simulink model "hexarotor_dynamic_model"  (Simulink 8.5)
settings: Solver=ode45  StartTime=0.0  StopTime=20  RelTol=1e-3
libraries: aerolib6dof2 x1
settings Model: Creator=flying  LastModifiedBy=flying
settings DataIOCC: ExternalInput=getinputstruct(op_trim1)  InitialState=getstatestruct(op_trim1)  LoadExternalInput=on  LoadInitialState=on  SignalLoggingSaveFormat=Dataset
settings OptimizationCC: ExpressionDepthLimit=128
settings DebuggingCC: UnderspecifiedInitializationDetection=Simplified  MergeDetectMultiDrivingBlocksExec=error  FcnCallInpInsideContextMsg=EnableAllAsError  StateNameClashWarn=none
settings GRTTargetCC: CombineOutputUpdateFcns=on  GRTInterface=off

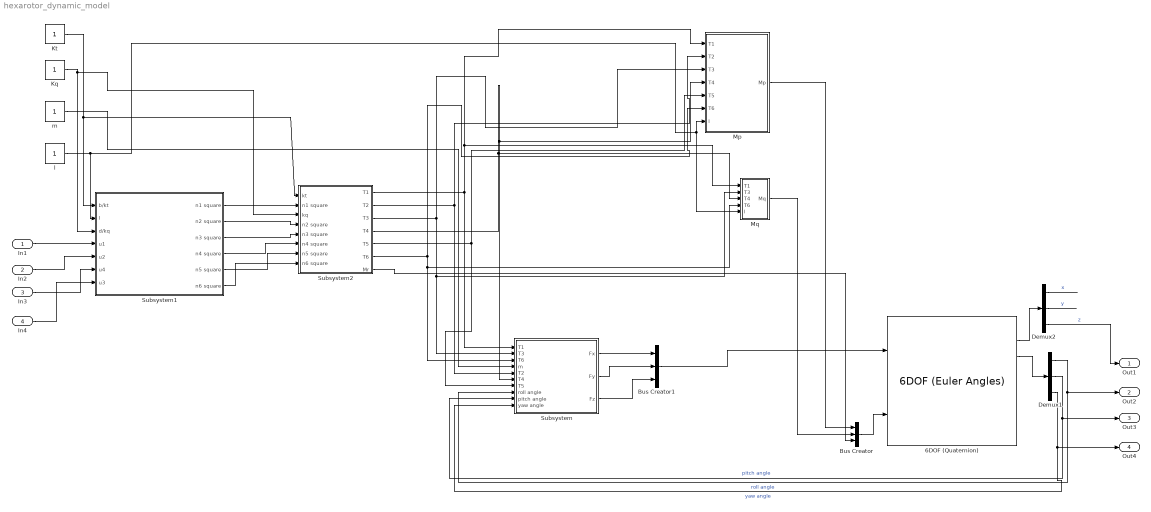
== system hexarotor_dynamic_model ==
  In1 : Inport
  In2 : Inport  Port=2
  In3 : Inport  Port=3
  In4 : Inport  Port=4
  6DOF (Quaternion) : aerolib6dof2/6DOF (Euler Angles)  units=Metric (MKS)  mtype=Fixed  rep=Quaternion  xme_0=[0 0 0]  Vm_0=[0 0 0]  eul_0=[0 0 0]  pm_0=[0 0 0]  mass_0=1.0  mass_e=0.5  mass_f=2.0  inertia=eye(3)  inertia_e=eye(3)  inertia_f=2*eye(3)  k_quat=1.0  vre_flag=on
  Bus Creator : BusCreator  Inputs=3
  Bus Creator1 : BusCreator  Inputs=3
  Demux1 : Demux  Outputs=3
  Demux2 : Demux  Outputs=3
  Kq : Constant
  Kt : Constant
  Mp : Subsystem
  Mq : Subsystem
  Subsystem : Subsystem
  Subsystem1 : Subsystem
  Subsystem2 : Subsystem
  l : Constant
  m : Constant
  Out1 : Outport
  Out2 : Outport  Port=2
  Out3 : Outport  Port=3
  Out4 : Outport  Port=4
  wires:
  6DOF (Quaternion)/3 -> Demux1/1
  l/1 -> Subsystem1/2(l), Mq/5(l), Mp/7(l)
  Mp/1(Mp) -> Bus Creator/1
  Mq/1(Mq) -> Bus Creator/2
  Subsystem2/2(T2) -> Mp/2(T2), Subsystem/5(T2)
  Subsystem2/4(T4) -> Subsystem/6(T4), Mp/4(T4), Mq/3(T4)
  Subsystem2/1(T1) -> Mp/1(T1), Mq/1(T1), Subsystem/1(T1)
  Subsystem2/6(T6) -> Subsystem/3(T6), Mq/4(T6), Mp/6(T6)
  Subsystem2/3(T3) -> Subsystem/2(T3), Mq/2(T3), Mp/3(T3)
  Subsystem2/5(T5) -> Subsystem/7(T5), Mp/5(T5)
  Kt/1 -> Subsystem1/1(b/kt), Subsystem2/1(kt)
  Kq/1 -> Subsystem1/3(d/kq), Subsystem2/3(kq)
  Subsystem2/7(Mr) -> Bus Creator/3
  Bus Creator/1 -> 6DOF (Quaternion)/2
  m/1 -> Subsystem/4(m)
  Demux1/1 -> Out2/1, Subsystem/8(roll angle)  "roll angle"
  Demux1/2 -> Out3/1, Subsystem/9(pitch angle)  "pitch angle"
  Demux1/3 -> Out4/1, Subsystem/10(yaw angle)  "yaw angle"
  Subsystem/1(Fx) -> Bus Creator1/1
  Subsystem/2(Fy) -> Bus Creator1/2
  Subsystem/3(Fz) -> Bus Creator1/3
  Bus Creator1/1 -> 6DOF (Quaternion)/1
  Subsystem1/1(n1 square) -> Subsystem2/2(n1 square)
  Subsystem1/2(n2 square) -> Subsystem2/4(n2 square)
  Subsystem1/3(n3 square) -> Subsystem2/5(n3 square)
  Subsystem1/4(n4 square) -> Subsystem2/6(n4 square)
  Subsystem1/5(n5 square) -> Subsystem2/7(n5 square)
  Subsystem1/6(n6 square) -> Subsystem2/8(n6 square)
  6DOF (Quaternion)/2 -> Demux2/1
  Demux2/1 -> ?  "x"
  Demux2/2 -> ?  "y"
  Demux2/3 -> Out1/1  "z"
  In1/1 -> Subsystem1/4(u1)
  In2/1 -> Subsystem1/5(u2)
  In3/1 -> Subsystem1/6(u4)
  In4/1 -> Subsystem1/7(u3)

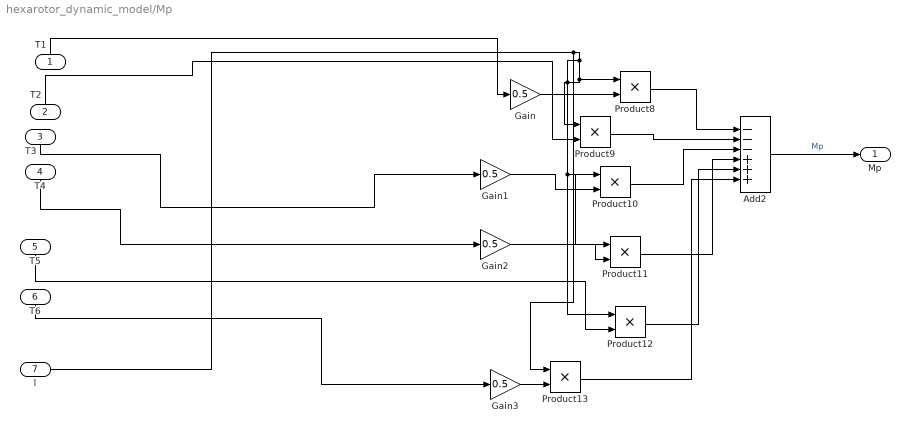
== system hexarotor_dynamic_model/Mp ==
  T1 : Inport
  T2 : Inport  Port=2
  T3 : Inport  Port=3
  T4 : Inport  Port=4
  T5 : Inport  Port=5
  T6 : Inport  Port=6
  l : Inport  Port=7
  Add2 : Sum  Inputs=---+++
  Gain{,1..3} (4 alike) : Gain  Gain=0.5
  Product{8..13} (6 alike) : Product
  Mp : Outport
  wires:
  T5/1 -> Product12/2
  T1/1 -> Gain/1
  T3/1 -> Gain1/1
  T6/1 -> Gain3/1
  T2/1 -> Product9/2
  T4/1 -> Gain2/1
  Add2/1 -> Mp/1  "Mp"
  Product9/1 -> Add2/2
  Product8/1 -> Add2/1
  Product10/1 -> Add2/3
  Gain3/1 -> Product13/2
  Product13/1 -> Add2/6
  Gain1/1 -> Product10/2
  Gain/1 -> Product8/2
  l/1 -> Product13/1, Product12/1, Product11/1, Product10/1, Product9/1, Product8/1
  Product12/1 -> Add2/5
  Gain2/1 -> Product11/2
  Product11/1 -> Add2/4

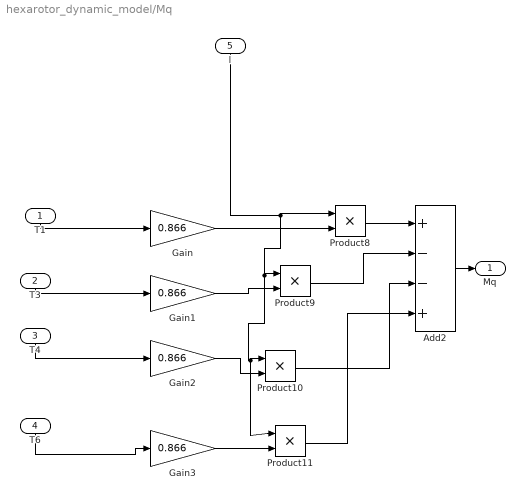
== system hexarotor_dynamic_model/Mq ==
  T1 : Inport
  T3 : Inport  Port=2
  T4 : Inport  Port=3
  T6 : Inport  Port=4
  l : Inport  Port=5
  Add2 : Sum  Inputs=+--+
  Gain{,1..3} (4 alike) : Gain  Gain=0.866
  Product{8..11} (4 alike) : Product
  Mq : Outport
  wires:
  Gain2/1 -> Product10/2
  Gain/1 -> Product8/2
  Gain1/1 -> Product9/2
  Product9/1 -> Add2/2
  Product10/1 -> Add2/3
  Product8/1 -> Add2/1
  Product11/1 -> Add2/4
  Gain3/1 -> Product11/2
  T1/1 -> Gain/1
  l/1 -> Product11/1, Product10/1, Product9/1, Product8/1
  T3/1 -> Gain1/1
  T6/1 -> Gain3/1
  Add2/1 -> Mq/1
  T4/1 -> Gain2/1

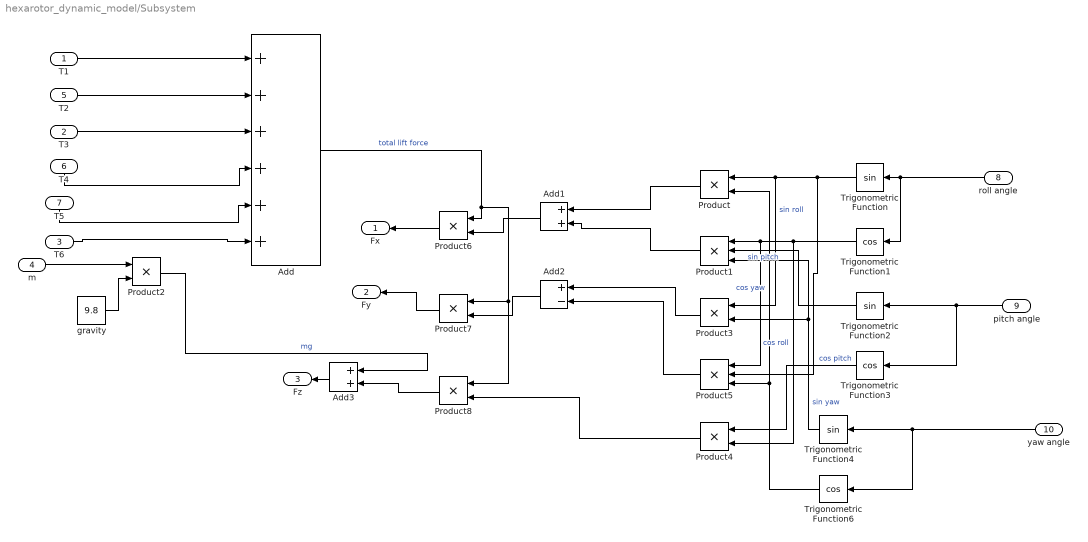
== system hexarotor_dynamic_model/Subsystem ==
  T1 : Inport
  T3 : Inport  Port=2
  T6 : Inport  Port=3
  m : Inport  Port=4
  T2 : Inport  Port=5
  T4 : Inport  Port=6
  T5 : Inport  Port=7
  roll angle : Inport  Port=8
  pitch angle : Inport  Port=9
  yaw angle : Inport  Port=10
  Add : Sum  Inputs=++++++
  Add1 : Sum
  Add2 : Sum  Inputs=+-
  Add3 : Sum
  Product{,2..4,6..8} (7 alike) : Product
  Product1 : Product  Inputs=3
  Product5 : Product  Inputs=3
  Trigonometric Function : Trigonometry
  Trigonometric Function1 : Trigonometry  Operator=cos
  Trigonometric Function2 : Trigonometry
  Trigonometric Function3 : Trigonometry  Operator=cos
  Trigonometric Function4 : Trigonometry
  Trigonometric Function6 : Trigonometry  Operator=cos
  gravity : Constant  Value=9.8
  Fx : Outport
  Fy : Outport  Port=2
  Fz : Outport  Port=3
  wires:
  Product7/1 -> Fy/1
  Product2/1 -> Add3/1  "mg"
  Trigonometric Function6/1 -> Product/2, Product5/3  "cos yaw"
  Product8/1 -> Add3/2
  Trigonometric Function/1 -> Product5/2, Product3/1, Product/1  "sin roll"
  Product1/1 -> Add1/2
  Product/1 -> Add1/1
  Trigonometric Function1/1 -> Product4/2, Product5/1, Product1/1  "cos roll"
  Trigonometric Function4/1 -> Product3/2, Product1/3  "sin yaw"
  Add2/1 -> Product7/2
  Add1/1 -> Product6/2
  Trigonometric Function2/1 -> Product1/2  "sin pitch"
  Product4/1 -> Product8/2
  Product3/1 -> Add2/1
  Product5/1 -> Add2/2
  Add/1 -> Product8/1, Product7/1, Product6/1  "total lift force"
  T1/1 -> Add/1
  T2/1 -> Add/2
  T6/1 -> Add/6
  T5/1 -> Add/5
  Add3/1 -> Fz/1
  T3/1 -> Add/3
  T4/1 -> Add/4
  yaw angle/1 -> Trigonometric Function6/1, Trigonometric Function4/1
  gravity/1 -> Product2/2
  m/1 -> Product2/1
  Product6/1 -> Fx/1
  Trigonometric Function3/1 -> Product4/1  "cos pitch"
  pitch angle/1 -> Trigonometric Function3/1, Trigonometric Function2/1
  roll angle/1 -> Trigonometric Function1/1, Trigonometric Function/1

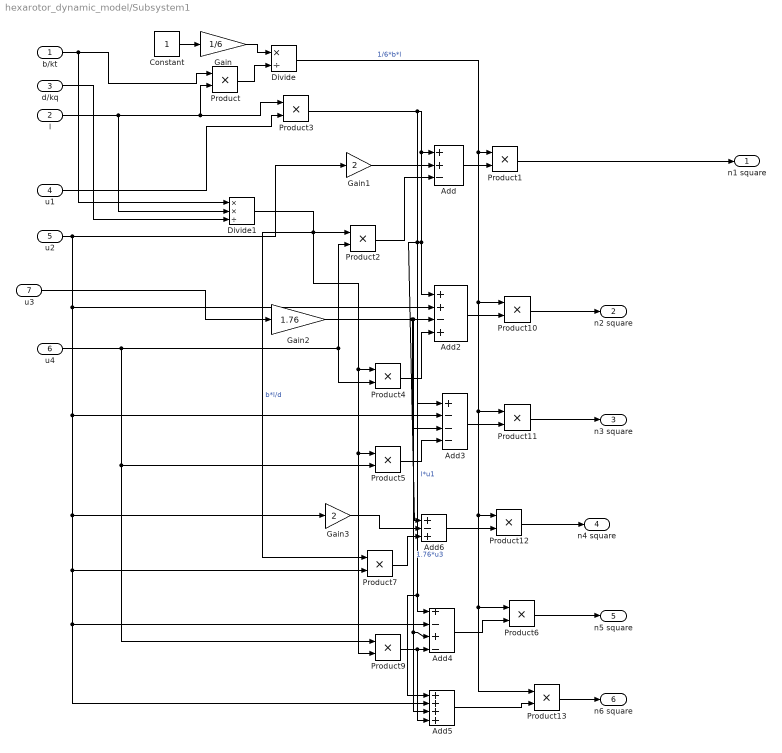
== system hexarotor_dynamic_model/Subsystem1 ==
  b/kt : Inport
  l : Inport  Port=2
  d/kq : Inport  Port=3
  u1 : Inport  Port=4
  u2 : Inport  Port=5
  u4 : Inport  Port=6
  u3 : Inport  Port=7
  Add : Sum  Inputs=++-
  Add2 : Sum  Inputs=++-+
  Add3 : Sum  Inputs=+---
  Add4 : Sum  Inputs=+-+-
  Add5 : Sum  Inputs=++++
  Add6 : Sum  Inputs=+-+
  Constant : Constant
  Divide : Product  Inputs=*/
  Divide1 : Product  Inputs=**/
  Gain : Gain  Gain=1/6
  Gain1 : Gain  Gain=2
  Gain2 : Gain  Gain=1.76
  Gain3 : Gain  Gain=2
  Product{,1..7,9..13} (13 alike) : Product
  n1 square : Outport
  n2 square : Outport  Port=2
  n3 square : Outport  Port=3
  n4 square : Outport  Port=4
  n5 square : Outport  Port=5
  n6 square : Outport  Port=6
  wires:
  d/kq/1 -> Divide1/3
  Gain3/1 -> Add6/2
  u1/1 -> Product3/2
  Divide1/1 -> Product9/2, Product5/1, Product4/1, Product7/1, Product2/1  "b*l/d"
  Add6/1 -> Product12/2
  Product12/1 -> n4 square/1
  Product7/1 -> Add6/3
  Add/1 -> Product1/2
  Product10/1 -> n2 square/1
  u2/1 -> Add5/2, Add4/2, Product7/2, Gain3/1, Add3/2, Add2/2, Gain1/1
  Product4/1 -> Add2/4
  u3/1 -> Gain2/1
  Product6/1 -> n5 square/1
  Add4/1 -> Product6/2
  Add5/1 -> Product13/2
  Add2/1 -> Product10/2
  Product3/1 -> Add5/1, Add4/1, Add6/1, Add3/1, Add2/1, Add/1  "l*u1"
  Gain1/1 -> Add/2
  u4/1 -> Product9/1, Product5/2, Product4/2, Product2/2
  Product1/1 -> n1 square/1
  Product5/1 -> Add3/4
  Gain2/1 -> Add5/3, Add4/3, Add2/3, Add3/3  "1.76*u3"
  Constant/1 -> Gain/1
  Product11/1 -> n3 square/1
  Divide/1 -> Product13/1, Product6/1, Product12/1, Product11/1, Product10/1, Product1/1  "1/6*b*l"
  Add3/1 -> Product11/2
  Gain/1 -> Divide/1
  l/1 -> Divide1/2, Product3/1, Product/2
  Product/1 -> Divide/2
  b/kt/1 -> Divide1/1, Product/1
  Product9/1 -> Add4/4, Add5/4
  Product13/1 -> n6 square/1
  Product2/1 -> Add/3

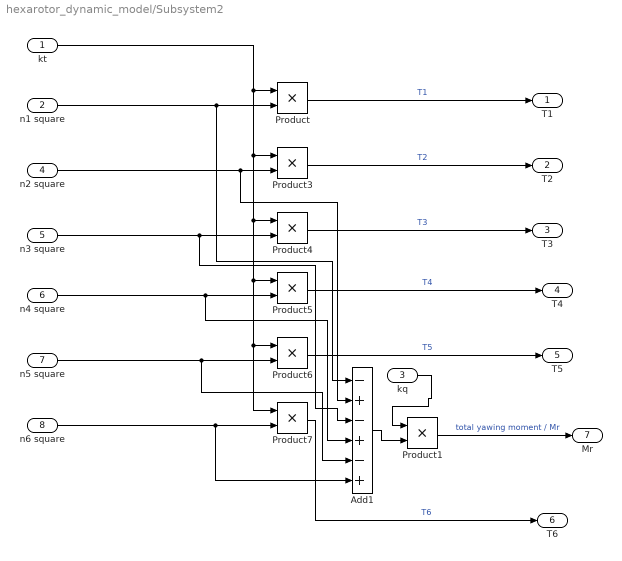
== system hexarotor_dynamic_model/Subsystem2 ==
  kt : Inport
  n1 square : Inport  Port=2
  kq : Inport  Port=3
  n2 square : Inport  Port=4
  n3 square : Inport  Port=5
  n4 square : Inport  Port=6
  n5 square : Inport  Port=7
  n6 square : Inport  Port=8
  Add1 : Sum  Inputs=-+-+-+
  Product{,1,3..7} (7 alike) : Product
  T1 : Outport
  T2 : Outport  Port=2
  T3 : Outport  Port=3
  T4 : Outport  Port=4
  T5 : Outport  Port=5
  T6 : Outport  Port=6
  Mr : Outport  Port=7
  wires:
  Product7/1 -> T6/1  "T6"
  n3 square/1 -> Add1/3, Product4/2
  n5 square/1 -> Add1/5, Product6/2
  Product3/1 -> T2/1  "T2"
  kq/1 -> Product1/1
  Product4/1 -> T3/1  "T3"
  n2 square/1 -> Add1/2, Product3/2
  n1 square/1 -> Add1/1, Product/2
  n4 square/1 -> Add1/4, Product5/2
  n6 square/1 -> Add1/6, Product7/2
  kt/1 -> Product7/1, Product6/1, Product5/1, Product4/1, Product3/1, Product/1
  Product1/1 -> Mr/1  "total yawing moment / Mr"
  Product6/1 -> T5/1  "T5"
  Product/1 -> T1/1  "T1"
  Product5/1 -> T4/1  "T4"
  Add1/1 -> Product1/2
